simulink model "DSS"  (Simulink 9.0)
settings: Solver=FixedStepDiscrete  StartTime=0.0  StopTime=10.0  FixedStep=0.100000  RelTol=1e-3  EnableMultiTasking=on
model workspace (MAT data in the model file):
  already_pp : num (value not decoded)
PreLoadFcn:
  | A = [1.303430790495574 0.435903405618026 ;0.581204540824034 1.739334196113600 ];
  | B = [0.510647680364470 ;0.500046006035811 ];
  | C = [1.000000000000000 5.000000000000000 ];
  | D = [2.000000000000000 ];
settings Model: SuppressorTable=22 serialization::archive 11 0 6 0 0 0 0 0  Creator=arnaud  LastModifiedBy=hbourbou
settings DataIOCC: LimitDataPoints=on  SaveFormat=Structure  SignalLoggingSaveFormat=ModelDataLogs
settings OptimizationCC: ExpressionDepthLimit=2147483647
settings DebuggingCC: AlgebraicLoopMsg=error  ArtificialAlgebraicLoopMsg=error  SolverPrmCheckMsg=warning  FcnCallInpInsideContextMsg=warning  StateNameClashWarn=warning
settings GRTTargetCC: GeneratePreprocessorConditionals=Disable all  CombineOutputUpdateFcns=off  GRTInterface=on
settings ConfigComp: CovSFcnEnable=off

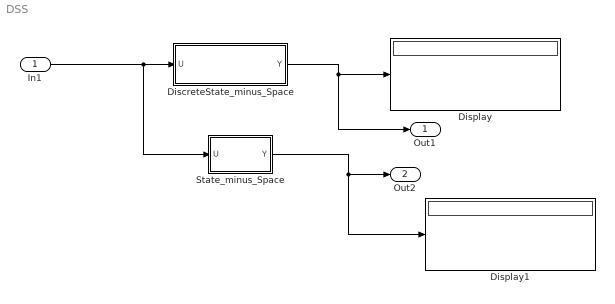
== system DSS ==
  In1 : Inport  OutDataTypeStr=double  PortDimensions=1
  DiscreteState_minus_Space : Subsystem  TreatAsAtomicUnit=on
  Display : Display
  Display1 : Display
  State_minus_Space : Subsystem  TreatAsAtomicUnit=on
  Out1 : Outport
  Out2 : Outport  Port=2
  wires:
  In1/1 -> State_minus_Space/1(U), DiscreteState_minus_Space/1(U)
  DiscreteState_minus_Space/1(Y) -> Out1/1, Display/1
  State_minus_Space/1(Y) -> Out2/1, Display1/1

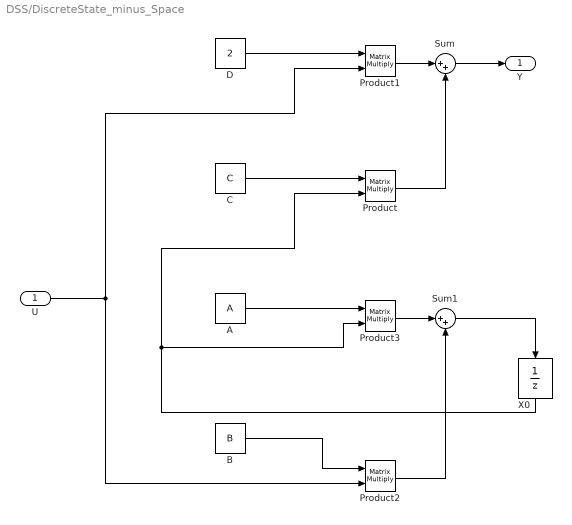
== system DSS/DiscreteState_minus_Space ==
  U : Inport  OutDataTypeStr=double  PortDimensions=1
  A : Constant  Value=A  VectorParams1D=off
  B : Constant  Value=B  VectorParams1D=off
  C : Constant  Value=C  VectorParams1D=off
  D : Constant  Value=2  VectorParams1D=off
  Product{,1..3} (4 alike) : Product  Multiplication=Matrix(*)
  Sum : Sum  Inputs=|++
  Sum1 : Sum  Inputs=|++
  X0 : UnitDelay  SampleTime=-1
  Y : Outport
  wires:
  Product3/1 -> Sum1/1
  A/1 -> Product3/1
  B/1 -> Product2/1
  Product2/1 -> Sum1/2
  Sum1/1 -> X0/1
  U/1 -> Product2/2, Product1/2
  D/1 -> Product1/1
  X0/1 -> Product3/2, Product/2
  C/1 -> Product/1
  Product1/1 -> Sum/1
  Product/1 -> Sum/2
  Sum/1 -> Y/1

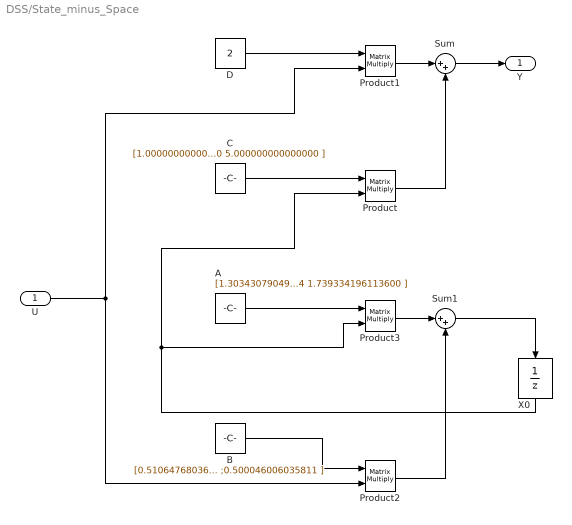
== system DSS/State_minus_Space ==
  U : Inport  OutDataTypeStr=double  PortDimensions=1
  A : Constant  Value=[1.303430790495574 0.435903405618026 ;0.581204540824034 1.739334196113600 ]  VectorParams1D=off
  B : Constant  Value=[0.510647680364470 ;0.500046006035811 ]  VectorParams1D=off
  C : Constant  Value=[1.000000000000000 5.000000000000000 ]  VectorParams1D=off
  D : Constant  Value=2  VectorParams1D=off
  Product{,1..3} (4 alike) : Product  Multiplication=Matrix(*)
  Sum : Sum  Inputs=|++
  Sum1 : Sum  Inputs=|++
  X0 : UnitDelay  InitialCondition=[0.000000000000000 ;0.000000000000000 ]  SampleTime=0.1
  Y : Outport
  wires:
  Product3/1 -> Sum1/1
  A/1 -> Product3/1
  B/1 -> Product2/1
  Product2/1 -> Sum1/2
  Sum1/1 -> X0/1
  U/1 -> Product2/2, Product1/2
  D/1 -> Product1/1
  X0/1 -> Product3/2, Product/2
  C/1 -> Product/1
  Product1/1 -> Sum/1
  Product/1 -> Sum/2
  Sum/1 -> Y/1
